simulink model "top_model"  (R2018b)
settings: Solver=VariableStepAuto  StartTime=0.0  StopTime=10.0  RelTol=1e-3  EnableMultiTasking=on
PostLoadFcn:
  | load('pcoeffs.mat');
  | load('rcoeffs.mat');
  | load('carparameters.mat');
  | 
  | %load('purelongdata.mat');
  | %load('purelongdataval.mat');
  | %load('purelatdata.mat');
  | %load('purelatdataval.mat');
  | load('combineddata.mat');
undefined symbols (not defined in the file): Id, m_car, reff
libraries: cstblocks x2, simulink x1
settings Model: Creator=The MathWorks, Inc.  LastModifiedBy=gdell
settings DataIOCC: LimitDataPoints=on
settings OptimizationCC: LifeSpan=inf
settings DebuggingCC: AllowSymbolicDim=off  SFUnexpectedBacktrackingDiag=warning  SFNoUnconditionalDefaultTransitionDiag=warning  SFExecutionAtInitializationDiag=none
settings ModelReferenceCC: PropagateSignalLabelsOutOfModel=off
settings SFSimCC: SimUseLocalCustomCode=off
settings RTWCC: RTWUseLocalCustomCode=off
settings CodeAppCC: StateflowObjectComments=on
settings GRTTargetCC: TargetLangStandard=C89/C90 (ANSI)
settings ConfigComp: CovMetricSettings=dw  CovHtmlReporting=on  CovSaveCumulativeToWorkspaceVar=on  CovSaveSingleToWorkspaceVar=on  CovExternalEMLEnable=off

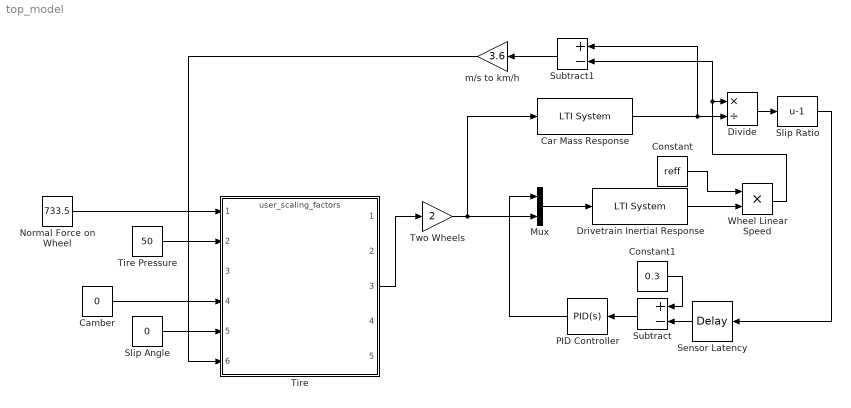
== system top_model ==
  "Camber " : Constant  Value=0
  Car Mass Response : cstblocks/LTI System  sys=ss(0, [1/m_car], 1, 0)  IC=[0.001]
  Constant : Constant  Value=reff
  Constant1 : Constant  Value=0.3
  Divide : Product  Inputs=*/
  "Drivetrain Inertial Response " : cstblocks/LTI System  sys=ss(0, [1/Id, -reff/Id], 1, 0)  IC=[0.0001]
  Mux : Mux  Inputs=2
  "Normal Force on Wheel " : Constant  Value=733.5
  PID Controller : simulink/Continuous/PID Controller  Controller=PID  Form=Parallel  TimeDomain=Continuous-time  SampleTime=-1  IntegratorMethod=Forward Euler  FilterMethod=Forward Euler  ControllerParametersSource=internal  P=500  I=7000  D=-0.0909966244971969  UseFilter=on  N=32.0990602641342  TunerSelectOption=Transfer Function Based (PID Tuner App)  ZeroCross=off  InitialConditionSource=internal  InitialConditionForIntegrator=0  InitialConditionForFilter=0  DifferentiatorICPrevScaledInput=0  ExternalReset=none  TrackingMode=off  Kt=1  LimitOutput=on  UpperSaturationLimit=8*240  LowerSaturationLimit=0  LinearizeAsGain=on  AntiWindupMode=none  Kb=1  POutMin=[]  POutMax=[]  IOutMin=[]  IOutMax=[]  DOutMin=[]  DOutMax=[]  NOutMin=[]  NOutMax=[]  SumOutMin=[]  SumOutMax=[]  SaturationOutMin=[]  SaturationOutMax=[]  PParamMin=[]  PParamMax=[]  IParamMin=[]  IParamMax=[]  DParamMin=[]  DParamMax=[]  NParamMin=[]  NParamMax=[]  KbParamMin=[]  KbParamMax=[]  KtParamMin=[]  KtParamMax=[]  KbOutMin=[]  KbOutMax=[]  KtOutMin=[]  KtOutMax=[]  IntegratorOutMin=[]  IntegratorOutMax=[]  FilterOutMin=[]  FilterOutMax=[]  SumI1OutMin=[]  SumI1OutMax=[]  SumI2OutMin=[]  SumI2OutMax=[]  SumI3OutMin=[]  SumI3OutMax=[]  SumI4OutMin=[]  SumI4OutMax=[]  SumDOutMin=[]  SumDOutMax=[]  DifferentiatorOutMin=[]  DifferentiatorOutMax=[]  FilterDiffOutCoefMin=[]  FilterDiffOutCoefMax=[]  ReciprocalOutMin=[]  ReciprocalOutMax=[]  SumDenOutMin=[]  SumDenOutMax=[]  SumNumOutMin=[]  SumNumOutMax=[]  DivideOutMin=[]  DivideOutMax=[]  IntegratorContinuousStateAttributes=''  IntegratorStateMustResolveToSignalObject=off  IntegratorRTWStateStorageClass=Auto  FilterContinuousStateAttributes=''  FilterStateMustResolveToSignalObject=off  FilterRTWStateStorageClass=Auto  ParallelPVariant=InternalParameters  IdealPVariant=Disabled  IVariant=InternalParameters  DVariant=InternalParameters  IntegratorVariant=Continuous  SatVariant=Enabled  AWVariant=Passthrough  PCopyVariant=Disabled  TRVariant=Disabled  FdbkBlocksVariant=Forward  IdealPFdbkVariant=Disabled  SatFdbkVariant=Disabled  DerivativeFilterVariant=ContFilter  NVariant=InternalParameters  NCopyVariant=Disabled  FilterICVariant=InternalICsFilter  IntegratorICVariant=InternalICs  ExternalResetVariant=Disabled  TRSumVariant=Passthrough  SumFdbkVariant=Disabled  SumVariant=Sum_PID
  "Sensor Latency " : TransportDelay  DelayTime=0.08
  "Slip Angle " : Constant  Value=0
  Slip Ratio : Bias  Bias=-1
  Subtract : Sum  Inputs=+-
  Subtract1 : Sum  Inputs=+-
  Tire : ModelReference  ModelNameDialog=user_scaling_factors.slx  SimulationMode=Normal  ModelReferenceVersion=1.174
  "Tire Pressure " : Constant  Value=50
  Two Wheels : Gain  Gain=2
  Wheel Linear Speed : Product
  m/s to km/h : Gain  Gain=3.6
  wires:
  "Sensor Latency "/1 -> Subtract/2
  Mux/1 -> "Drivetrain Inertial Response "/1
  Constant1/1 -> Subtract/1
  m/s to km/h/1 -> Tire/6
  Two Wheels/1 -> Car Mass Response/1, Mux/2
  Subtract/1 -> PID Controller/1
  "Tire Pressure "/1 -> Tire/2
  Divide/1 -> Slip Ratio/1
  PID Controller/1 -> Mux/1
  "Camber "/1 -> Tire/4
  "Drivetrain Inertial Response "/1 -> Wheel Linear Speed/2
  Slip Ratio/1 -> "Sensor Latency "/1
  "Slip Angle "/1 -> Tire/5
  "Normal Force on Wheel "/1 -> Tire/1
  Wheel Linear Speed/1 -> Subtract1/2, Divide/1
  Constant/1 -> Wheel Linear Speed/1
  Car Mass Response/1 -> Subtract1/1, Divide/2
  Tire/3 -> Two Wheels/1
  Subtract1/1 -> m/s to km/h/1
